simulink model "ex7_model"  (R2015b)
settings: Solver=VariableStepAuto  StartTime=0.0  StopTime=10.0  RelTol=1e-3
settings Model: Creator=Tomáš  LastModifiedBy=Tomáš

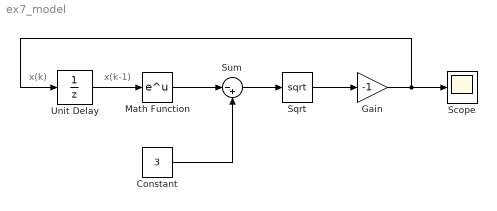
== system ex7_model ==
  note: x(k-1)
  note: x(k)
  Constant : Constant  Value=3
  Gain : Gain  Gain=-1
  Math Function : Math  SaturateOnIntegerOverflow=on
  Scope : Scope
  Sqrt : Sqrt  SaturateOnIntegerOverflow=on
  Sum : Sum  Inputs=|-+
  Unit Delay : UnitDelay  InitialCondition=-2  SampleTime=0.1
  wires:
  Unit Delay/1 -> Math Function/1
  Math Function/1 -> Sum/1
  Constant/1 -> Sum/2
  Sum/1 -> Sqrt/1
  Sqrt/1 -> Gain/1
  Gain/1 -> Scope/1, Unit Delay/1
